simulink model "PEAKDETECTOR4"  (R2018b)
settings: Solver=FixedStepDiscrete  StartTime=0.0  StopTime=150  RelTol=1e-3  EnableMultiTasking=on
undefined symbols (not defined in the file): fdesignblkfcn, gcbh
libraries: simulink x1, dspfdesign x1, dspsrcs4 x1, dspsigops x1
settings Model: ExtModeTrigDuration=2  Creator=Alex  LastModifiedBy=xpart
settings OptimizationCC: EnhancedBackFolding=on  PassReuseOutputArgsAs=Individual arguments  MaxStackSize=64  OptimizeBlockOrder=speed  DifferentSizesBufferReuse=on
settings DebuggingCC: ParameterTunabilityLossMsg=error
settings HardwareCC: ProdBitPerInt=16  ProdBitPerPointer=16  ProdBitPerSizeT=16  ProdBitPerPtrDiffT=16  ProdLargestAtomicFloat=None  ProdWordSize=8  ProdHWDeviceType=Atmel->AVR  UseEmbeddedCoderFeatures=off
settings SFSimCC: MATLABDynamicMemAlloc=off
settings RTWCC: SystemTargetFile=ert.tlc  HardwareBoard=Arduino Mega 2560  TemplateMakefile=ert_default_tmf  GenerateReport=on  Toolchain=Arduino AVR  BuildConfiguration=Faster Runs  IncludeHyperlinkInReport=on  LaunchReport=on  GenerateTraceInfo=on  GenerateTraceReport=on  GenerateTraceReportSl=on  GenerateTraceReportSf=on  GenerateTraceReportEml=on
settings CodeAppCC: ForceParamTrailComments=on  OperatorAnnotations=on  SimulinkDataObjDesc=on  SFDataObjDesc=on  InsertBlockDesc=on
settings ERTTargetCC: SupportContinuousTime=on  SupportNonInlinedSFcns=on  SupportVariableSizeSignals=on  ExtMode=on  ExtModeMexArgs='127.0.0.1' 0 17725  ERTSrcFileBannerTemplate=codertarget_code_template.cgt  ERTHdrFileBannerTemplate=codertarget_code_template.cgt  ERTDataSrcFileTemplate=codertarget_code_template.cgt  ERTDataHdrFileTemplate=codertarget_code_template.cgt

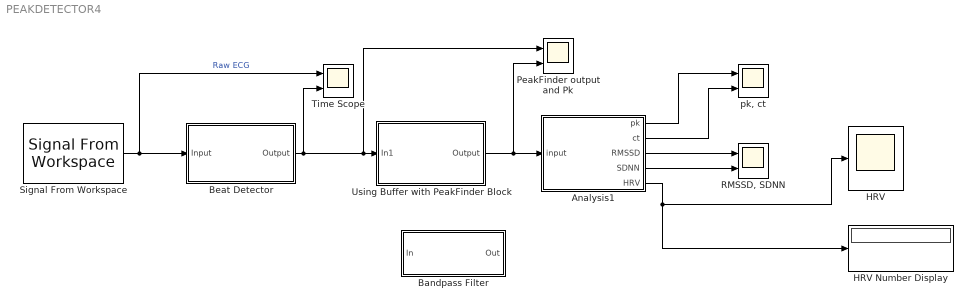
== system PEAKDETECTOR4 ==
  Analysis1 : MATLAB Function  TreatAsAtomicUnit=on
  Bandpass Filter : Subsystem  DialogController=fdesignblkfcn  InitFcn=fdesignblkfcn(gcbh, {'InitFcn'});  mask(Bandpass Filter){}
      mask help: Design a bandpass filter
      settings: CopyFcn=fdesignblkfcn(gcbh, {'CopyFcn'});
      mask Help: helpview(mapfilelocation('dsp'), 'dspbandpassfilter');
      mask Display: disp('Bandpass');
  Beat Detector : Subsystem
  HRV : Scope
  HRV Number Display : Display
      settings: Decimation=5
  PeakFinder output and Pk : Scope  NumInputPorts=2
  "RMSSD, SDNN" : Scope  NumInputPorts=2
  Signal From Workspace : dspsrcs4/Signal From Workspace  X=y  Ts=.004  nsamps=1  OutputAfterFinalValue=Setting to zero  ignoreOrWarnInputAndFrameLengths=off  OutputFrames=off
  Time Scope : Scope  NumInputPorts=2
  "Using Buffer with PeakFinder Block " : Subsystem
  "pk, ct" : Scope  NumInputPorts=2
  wires:
  "Using Buffer with PeakFinder Block "/1(Output) -> PeakFinder output and Pk/2, Analysis1/1(input)
  Analysis1/1(pk) -> "pk, ct"/1
  Analysis1/2(ct) -> "pk, ct"/2
  Analysis1/3(RMSSD) -> "RMSSD, SDNN"/1
  Beat Detector/1(Output) -> Time Scope/2, PeakFinder output and Pk/1, "Using Buffer with PeakFinder Block "/1(In1)
  Analysis1/4(SDNN) -> "RMSSD, SDNN"/2
  Analysis1/5(HRV) -> HRV Number Display/1, HRV/1
  Signal From Workspace/1 -> Beat Detector/1(Input), Time Scope/1  "Raw ECG"

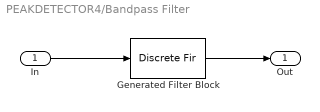
== system PEAKDETECTOR4/Bandpass Filter ==
  In : Inport
  Generated Filter Block : DiscreteFir  Tag=BlockMethodSubSystem  Coefficients=[-0.0008992291487744296 0.0016414518747943749 0.0031352071842225397 -0.0040707550828814922 -0.0063731852227904111 0.0074874286806090491 0.0098354319566295711 -0.010189316513446216 -0.011302794465874122 0.0096929185841818435 0.0079428653987464216 -0.0031368247881221642 0.0028299878877943137 -0.011508674243001471 -0.022080136219461581 0.034245325424507672 0.048356661648905473 -0.062355369169884239 -0.077503478162593897 0.090687768153125653 0.10353171105844157 -0.11297860084229834 -0.12035866024978455 0.12379360801539134 0.12379360801539134 -0.12035866024978455 -0.11297860084229834 0.10353171105844157 0.090687768153125653 -0.077503478162593897 -0.062355369169884239 0.048356661648905473 0.034245325424507672 -0.022080136219461581 -0.011508674243001471 0.0028299878877943137 -0.0031368247881221642 0.0079428653987464216 0.0096929185841818435 -0.011302794465874122 -0.010189316513446216 0.0098354319566295711 0.0074874286806090491 -0.0063731852227904111 -0.0040707550828814922 0.0031352071842225397 0.0016414518747943749 -0.0008992291487744296]  InputProcessing=Columns as channels (frame based)
  Out : Outport
  wires:
  In/1 -> Generated Filter Block/1
  Generated Filter Block/1 -> Out/1

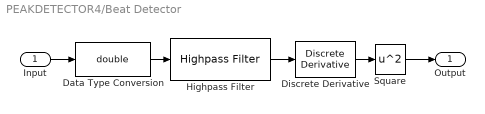
== system PEAKDETECTOR4/Beat Detector ==
  Input : Inport
  Data Type Conversion : DataTypeConversion  OutDataTypeStr=double
  "Discrete Derivative " : simulink/Discrete/Discrete Derivative  gainval=0.1  ICPrevScaledInput=0.0  OutMin=[]  OutMax=[]  OutDataType=fixdt(1, 16)  OutScaling=2^-10  DoSatur=off
  Highpass Filter : dspfdesign/Highpass Filter  FilterType=IIR  DesignForMinimumOrder=on  FilterOrder=50  StopbandFrequency=.05  PassbandFrequency=2  StopbandAttenuation=40  PassbandRipple=0.5  InheritSampleRate=off  SampleRate=250  SimulateUsing=Interpreted execution  roundingMode=Floor  coeffsDataTypeStr=fixdt(1,16)
      settings: SourceProductName=DSP System Toolbox
  Square : Math  Operator=square  SaturateOnIntegerOverflow=on
  Output : Outport
  wires:
  "Discrete Derivative "/1 -> Square/1
  Data Type Conversion/1 -> Highpass Filter/1
  Highpass Filter/1 -> "Discrete Derivative "/1
  Input/1 -> Data Type Conversion/1
  Square/1 -> Output/1

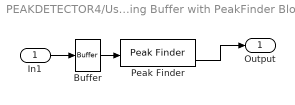
== system PEAKDETECTOR4/Using Buffer with PeakFinder Block  ==
  In1 : Inport
  Buffer : Buffer  N=3  V=2  OutputFrames=off
  Peak Finder : dspsigops/Peak Finder  polarity=Maxima  outputIdx=off  outputVal=on  maxPeaks=1  NoiseDistinguish=off  thresh=100000000  roundingMode=Floor  overflowMode=off
      settings: SourceProductName=DSP System Toolbox  SourceProductBaseCode=DS  allowOverrides=off
  Output : Outport
  wires:
  In1/1 -> Buffer/1
  Buffer/1 -> Peak Finder/1
  Peak Finder/2 -> Output/1

== matlab function PEAKDETECTOR4/Analysis1 ==
  data: input input; pk output; ct output; RMSSD output; SDNN output; HRV output
function [pk, ct, RMSSD, SDNN, HRV] = untitled2(input) 
%This function will examine the output of the PEAKFINDER block in simulink
%to calculate HRV. This system uses a Sampling Rate of 250 Hz, and where:
%       pk = the value of the peak that meets the peak requirements
%       ct = the time duration of a detected RR interval
%       HRV = SDNN/RMSSD
%
% *Persistent RMSSD, SDNN, and HRV are defined separately from the outputs 
%  of this function, solely so that there is an output for these values
%  even when there is no RR interval detected. 


persistent counter;     %Time Counter
persistent N;           %Number of intervals
persistent int1;        %First RR interval
persistent int2;        %Second RR interval
persistent pRMSSD;      %Persistent RMSSD *
persistent pSumRMSSD;   %Used for summation part of the RMSSD formula


persistent meanIntSum;
persistent meanInt;
persistent pSDNNSum;
persistent pSDNN;       %Persistent SDNN  *

persistent pHRV;        %Persistent HRV   *




minpeakdist = 0.6;              %Minimum distance betweek peaks
threshold = 600000;               %Threshold for peaks


% initializing persistent variables
if isempty(counter)
    int1 = 0;
    int2 = 0;
    N = 0;
    counter = 0; %starting at second sample where t = 0.008s
    pSumRMSSD = 0;
    pRMSSD = 0;
    RMSSD = 0;
    SDNN = 0;

    pSDNN = 0;
    meanIntSum = 0;
    meanInt = 0;
    pSDNNSum = 0;
    pHRV = 0;
    
end

%IF PEAK DETECTED: 
if input > threshold && counter > minpeakdist 
    pk = input;         %1. OUTPUT: Value of peak detected
    ct = counter;       %2. OUTPUT: time count
    N = N + 1;          %3. Increase peak count
    RMSSD = pRMSSD;     %4. OUTPUT: RMSSD as previously calculated
    SDNN = pSDNN; 
    
    
    %WHEN ONLY 1 PEAK DETECTED:  
    
    if N == 1              %First peak sets up measurement of RR intervals
        RMSSD = pRMSSD;    %OUTPUT: RMSSD as previously defined (0 here)
        SDNN = pSDNN;
        counter = 0;       %Reset the time counter
    end
    
    %WHEN 2 PEAKS DETECTED: 
    
    if N == 2               %We now have the first interval between 2 peaks
        
        %FOR SDNN:
        meanIntSum = meanIntSum + ct;
        meanInt = (1/(N-1))*meanIntSum;
        pSDNNSum = pSDNNSum + (ct - meanInt)^2;
        pSDNN = sqrt((1/(N-1)) * pSDNNSum);
        SDNN = pSDNN;                            %OUTPUT: SDNN
        
        
        %FOR RMSSD:
        int1 = ct;         %Define the first interval for RMSSD calculation
        RMSSD = pRMSSD;     %Still should be 0 in this case
        
        counter = 0;
    end
    
    if N >= 3    %3 Peaks gives us 2 interval calculate RMSSD
            
        %FOR SDNN:
        meanIntSum = meanIntSum + ct;
        meanInt = (1/(N-1))*meanIntSum;
        pSDNNSum = pSDNNSum + (ct - meanInt)^2;
        pSDNN = sqrt((1/(N-1)) * pSDNNSum);
        SDNN = pSDNN;                            %OUTPUT: SDNN
        
        %FOR RMSSD:
        int2 = counter;                          %Set the value for the second interval
        pSumRMSSD = pSumRMSSD + (int2 - int1)^2; %Calculate Summation in RMSSD formula
        pRMSSD = sqrt((1/(N-2))*pSumRMSSD);      %Calculate persistent RMSSD
        RMSSD = pRMSSD;                          %OUTPUT: RMSSD
        int1 = int2;                             %Swap the interval values 
        counter = 0;                             %Set time counter back to 0
    end
    
    pHRV = SDNN/RMSSD;
    HRV = pHRV;
    
%WHEN NO PEAK DETECTED:

else
    counter = counter + .004;   %1. Add to the time counter
    ct = counter;               %2. OUTPUT: The time counter value
    pk = 0;                     %3. OUTPUT: No Peak Value
    RMSSD = pRMSSD;             %4. OUTPUT THE RMSSD of last peak
    SDNN = pSDNN;               %5. Output the SDNN of last peak
    HRV = pHRV;                 %6. Output HRV of last peak
                                
end

end
